simulink model "PID3"  (R2021a)
settings: Solver=VariableStepAuto  StartTime=0.0  StopTime=5000  RelTol=1e-3
settings Model: Creator=mengw  LastModifiedBy=ximnic.Leo

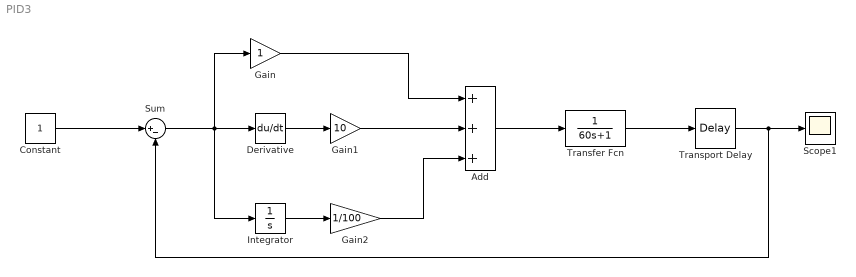
== system PID3 ==
  Add : Sum  Inputs=+++
  Constant : Constant
  Derivative : Derivative
  Gain : Gain
  Gain1 : Gain  Gain=10
  Gain2 : Gain  Gain=1/100
  Integrator : Integrator
  Scope1 : Scope
  Sum : Sum  Inputs=|+-
  Transfer Fcn : TransferFcn  Denominator=[60 1]
  Transport Delay : TransportDelay  DelayTime=80
  wires:
  Constant/1 -> Sum/1
  Sum/1 -> Integrator/1, Derivative/1, Gain/1
  Gain/1 -> Add/1
  Derivative/1 -> Gain1/1
  Integrator/1 -> Gain2/1
  Add/1 -> Transfer Fcn/1
  Transfer Fcn/1 -> Transport Delay/1
  Transport Delay/1 -> Sum/2, Scope1/1
  Gain2/1 -> Add/3
  Gain1/1 -> Add/2
